simulink model "Decoupler"  (R2015b)
settings: Solver=FixedStepAuto  StartTime=0.0  StopTime=inf  RelTol=1e-3
libraries: robotlib x5
settings Model: Creator=erik  LastModifiedBy=rasrack
settings OptimizationCC: ZeroExternalMemoryAtStartup=off  OptimizeModelRefInitCode=on  MaxStackSize=64
settings HardwareCC: ProdBitPerPointer=32  ProdLargestAtomicFloat=None  ProdIntDivRoundTo=Undefined  ProdEndianess=Unspecified  ProdWordSize=32  ProdHWDeviceType=Generic->Unspecified (assume 32-bit Generic)
settings RTWCC: SystemTargetFile=ert.tlc  TemplateMakefile=ert_default_tmf  Description=Embedded Coder  Toolchain=Catkin  TargetLang=C++
settings CodeAppCC: IgnoreCustomStorageClasses=off
settings ERTTargetCC: MultiInstanceERTCode=on  CodeInterfacePackaging=C++ class  SupportVariableSizeSignals=on  RootIOFormat=Structure reference

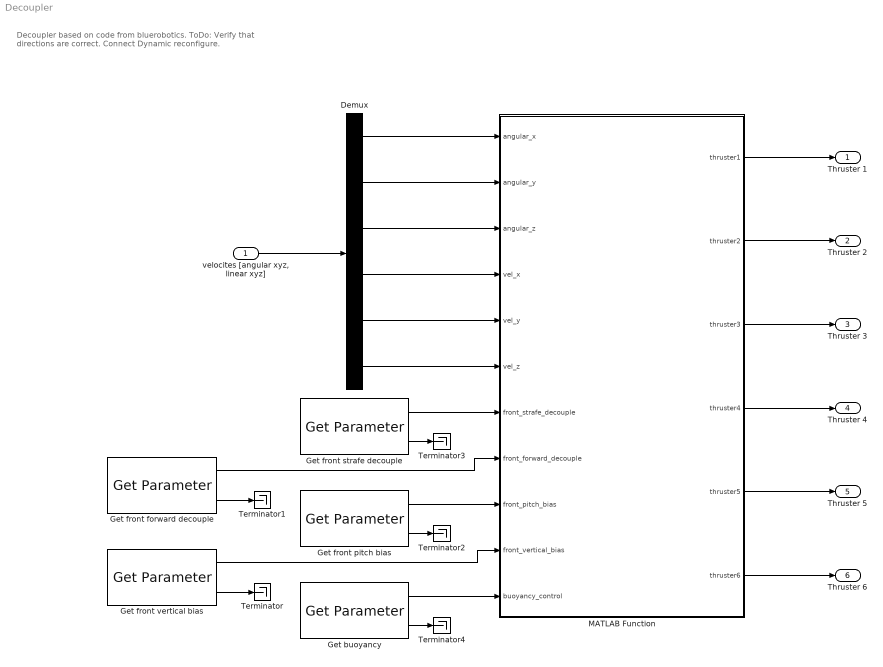
== system Decoupler ==
  note: Decoupler based on code from bluerobotics.
      | ToDo:
      | Verify that directions are correct.
      | Connect Dynamic reconfigure.
  "velocites [angular xyz, linear xyz]    " : Inport
  Demux : Demux  Outputs=6
  Get buoyancy : robotlib/Get Parameter  SourceLibraryInfo=This block requires Robotics System Toolbox  ParameterSource=Select from ROS network  ParameterName=/matlab_controller/buoyancy_control  ParameterType=double  ParameterInitialValue=0.0  SampleTime=-1  ShowErrorCodeOutput=on  ModelName=Decoupler  BlockId=ParamGet_Decoupler_14
  Get front forward decouple : robotlib/Get Parameter  SourceLibraryInfo=This block requires Robotics System Toolbox  ParameterSource=Select from ROS network  ParameterName=/matlab_controller/front_forward_decouple  ParameterType=double  ParameterInitialValue=0.0  SampleTime=-1  ShowErrorCodeOutput=on  ModelName=Decoupler  BlockId=ParamGet_Decoupler_18
  Get front pitch bias : robotlib/Get Parameter  SourceLibraryInfo=This block requires Robotics System Toolbox  ParameterSource=Select from ROS network  ParameterName=/matlab_controller/front_pitch_bias  ParameterType=double  ParameterInitialValue=0.0  SampleTime=-1  ShowErrorCodeOutput=on  ModelName=Decoupler  BlockId=ParamGet_Decoupler_17
  Get front strafe decouple : robotlib/Get Parameter  SourceLibraryInfo=This block requires Robotics System Toolbox  ParameterSource=Select from ROS network  ParameterName=/matlab_controller/front_strafe_decouple  ParameterType=double  ParameterInitialValue=0.0  SampleTime=-1  ShowErrorCodeOutput=on  ModelName=Decoupler  BlockId=ParamGet_Decoupler_19
  Get front vertical bias : robotlib/Get Parameter  SourceLibraryInfo=This block requires Robotics System Toolbox  ParameterSource=Select from ROS network  ParameterName=/matlab_controller/front_vertical_bias  ParameterType=double  ParameterInitialValue=0.0  SampleTime=-1  ShowErrorCodeOutput=on  ModelName=Decoupler  BlockId=ParamGet_Decoupler_16
  MATLAB Function : MATLAB Function  TreatAsAtomicUnit=on
  Terminator{,1..4} (5 alike) : Terminator
  Thruster 1 : Outport
  Thruster 2 : Outport  Port=2
  Thruster 3 : Outport  Port=3
  Thruster 4 : Outport  Port=4
  Thruster 5 : Outport  Port=5
  Thruster 6 : Outport  Port=6
  wires:
  MATLAB Function/1(thruster1) -> Thruster 1/1
  Get buoyancy/1 -> MATLAB Function/11(buoyancy_control)
  Get front vertical bias/1 -> MATLAB Function/10(front_vertical_bias)
  Get front pitch bias/1 -> MATLAB Function/9(front_pitch_bias)
  Get front forward decouple/1 -> MATLAB Function/8(front_forward_decouple)
  Get front strafe decouple/1 -> MATLAB Function/7(front_strafe_decouple)
  Demux/5 -> MATLAB Function/5(vel_y)
  Demux/6 -> MATLAB Function/6(vel_z)
  Demux/4 -> MATLAB Function/4(vel_x)
  Demux/3 -> MATLAB Function/3(angular_z)
  Demux/2 -> MATLAB Function/2(angular_y)
  Demux/1 -> MATLAB Function/1(angular_x)
  MATLAB Function/6(thruster6) -> Thruster 6/1
  MATLAB Function/5(thruster5) -> Thruster 5/1
  MATLAB Function/4(thruster4) -> Thruster 4/1
  MATLAB Function/3(thruster3) -> Thruster 3/1
  MATLAB Function/2(thruster2) -> Thruster 2/1
  Get front vertical bias/2 -> Terminator/1
  Get front forward decouple/2 -> Terminator1/1
  Get front pitch bias/2 -> Terminator2/1
  Get front strafe decouple/2 -> Terminator3/1
  Get buoyancy/2 -> Terminator4/1
  "velocites [angular xyz, linear xyz]    "/1 -> Demux/1

== matlab function Decoupler/MATLAB Function ==
  data: angular_x input; thruster1 output; angular_y input; angular_z input; vel_x input; vel_y input; vel_z input; front_strafe_decouple input; front_forward_decouple input; front_pitch_bias input; front_vertical_bias input; buoyancy_control input; thruster2 output; thruster3 output; thruster4 output; thruster5 output; thruster6 output
function [thruster1,thruster2,thruster3,thruster4,thruster5,thruster6] =...
    basicdecouple(angular_x,angular_y,angular_z,vel_x,vel_y,vel_z,...
    front_strafe_decouple,front_forward_decouple,front_pitch_bias,...
    front_vertical_bias,buoyancy_control)

% Vertical Left thruster (VL)
thruster1 =...
    angular_x...
    -front_forward_decouple*vel_x...
    -front_strafe_decouple*vel_y...
    -front_pitch_bias*angular_y...
    +front_vertical_bias*vel_z...
    +buoyancy_control; 


% Vertical Back thruster (VB)
thruster2 =...
    front_forward_decouple * vel_x...
    +angular_y...
    +vel_z...
    +buoyancy_control; 


thruster3 =...
    -angular_x...
    -front_forward_decouple * vel_x+...
    front_strafe_decouple*vel_y...
    -front_pitch_bias*angular_y...
    +front_vertical_bias * vel_z...
    +buoyancy_control;

 %Forward Left (FL)
thruster4 =...
    -angular_z...
    + vel_x;
thruster5 = vel_y; % LATeral (LAT)

% Forward Right (FR)
thruster6 =...
    angular_z...
    + vel_x;

end
